simulink model "bms_final_sims_06"  (R2017b)
settings: Solver=VariableStepAuto  StartTime=0.0  StopTime=600  MaxStep=1e-4  RelTol=1e-3
undefined symbols (not defined in the file): DiscIntNeverNeededParam, Ion, Lithium, Ts_Control
libraries: powerlib x61, simulink x20, powerlib_meascontrol x3, simulink_extras x1, electricdrivelib x1
(part 1 of 2)
settings Model: SimulationMode=accelerator  Creator=Saagar  LastModifiedBy=student
settings OptimizationCC: EfficientMapNaN2IntZero=off
settings HardwareCC: TargetBitPerPointer=64  TargetBitPerSizeT=64  TargetBitPerPtrDiffT=64  TargetLongLongMode=on  TargetIntDivRoundTo=Zero  TargetEndianess=LittleEndian  TargetWordSize=64  TargetHWDeviceType=MATLAB Host  ProdEqTarget=off
settings CodeAppCC: MaxIdLength=128
settings GRTTargetCC: TargetLangStandard=C89/C90 (ANSI)  CombineOutputUpdateFcns=off  GRTInterface=on

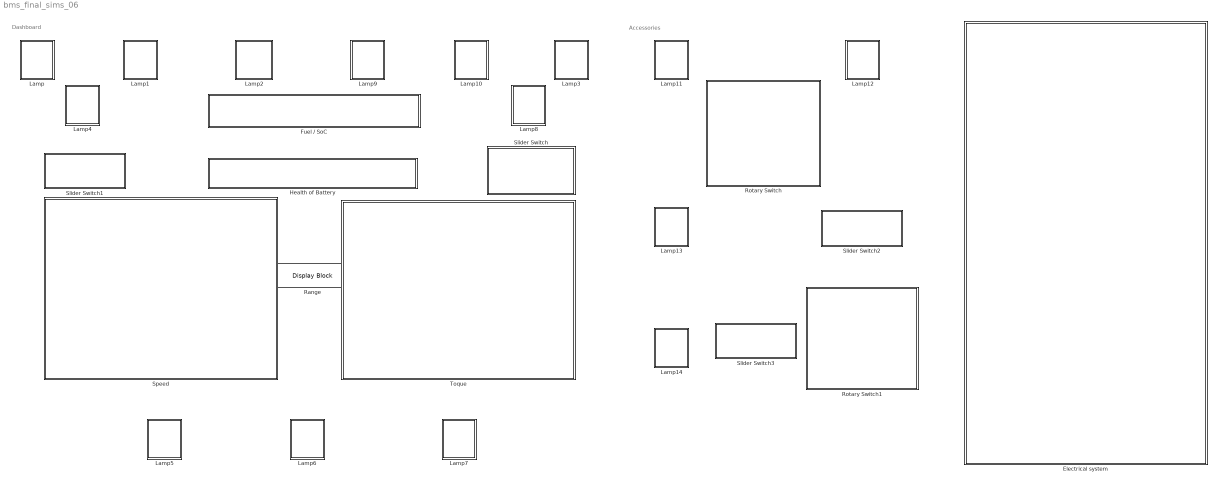
== system bms_final_sims_06 ==
  note: Accessories
  note: Dashboard
  Electrical system : Subsystem
  Fuel / SoC : Subsystem  DialogController=hmiCreateDDGDialog  IsWebBlock=on  mask(MWDashboardBlock){webBlockId=33162039-c99d-4f1a-a565-4d682c8cdccd, webBlockType=lineargauge, ShowInLibBrowser=on, ShowInitialText=on, HMISrcModelName=bms_final_sims_06}
      mask prompts: webBlockId "WebBlock Id"; webBlockType "WebBlock Type"; HMISrcModelName "Source Model"
      mask help: SimulinkHMI:dialogs:LinearGaugeDialogDesc
      mask Help: helpview([docroot '/mapfiles/simulink.map'], 'hmi_linear_gauge')
      mask Display:
      | if strcmp(get_param(bdroot(gcb),'BlockDiagramType'), 'library')
      |     image([(matlabroot) '/toolbox/simulink/hmi/icons/LinearGauge.png']);
      | end
  Health of Battery : Subsystem  DialogController=hmiCreateDDGDialog  IsWebBlock=on  mask(MWDashboardBlock){webBlockId=8809f0b6-5e37-4dfb-af47-87218bc99b36, webBlockType=lineargauge, ShowInLibBrowser=on, ShowInitialText=on, HMISrcModelName=bms_final_sims_06}
      mask prompts: webBlockId "WebBlock Id"; webBlockType "WebBlock Type"; HMISrcModelName "Source Model"
      mask help: SimulinkHMI:dialogs:LinearGaugeDialogDesc
      mask Help: helpview([docroot '/mapfiles/simulink.map'], 'hmi_linear_gauge')
      mask Display:
      | if strcmp(get_param(bdroot(gcb),'BlockDiagramType'), 'library')
      |     image([(matlabroot) '/toolbox/simulink/hmi/icons/LinearGauge.png']);
      | end
  Lamp : Subsystem  DialogController=hmiCreateDDGDialog  IsWebBlock=on  mask(MWDashboardBlock){webBlockId=60202423-3a17-48a5-95f7-77e0dff5e21e, webBlockType=lamp, ShowInLibBrowser=on, ShowInitialText=on, HMISrcModelName=bms_final_sims_06}
      mask prompts: webBlockType "WebBlock Type"; HMISrcModelName "Source Model"
      mask help: SimulinkHMI:dialogs:LampDialogDesc
      mask Help: helpview([docroot '/mapfiles/simulink.map'], 'hmi_lamp')
      mask Display:
      | if strcmp(get_param(bdroot(gcb),'BlockDiagramType'), 'library')
      |     image([(matlabroot) '/toolbox/simulink/hmi/icons/Lamp.png']);
      | end
  Lamp1 : Subsystem  DialogController=hmiCreateDDGDialog  IsWebBlock=on  mask(MWDashboardBlock){webBlockId=b772b617-bcd0-40f5-b9ce-808a282dbb2f, webBlockType=lamp, ShowInLibBrowser=on, ShowInitialText=on, HMISrcModelName=bms_final_sims_06}
      mask prompts: webBlockType "WebBlock Type"; HMISrcModelName "Source Model"
      mask help: SimulinkHMI:dialogs:LampDialogDesc
      mask Help: helpview([docroot '/mapfiles/simulink.map'], 'hmi_lamp')
      mask Display:
      | if strcmp(get_param(bdroot(gcb),'BlockDiagramType'), 'library')
      |     image([(matlabroot) '/toolbox/simulink/hmi/icons/Lamp.png']);
      | end
  Lamp10 : Subsystem  DialogController=hmiCreateDDGDialog  IsWebBlock=on  mask(MWDashboardBlock){webBlockId=5d6d0afe-77fe-451f-a78c-39b64214a0af, webBlockType=lamp, ShowInLibBrowser=on, ShowInitialText=on, HMISrcModelName=bms_final_sims_06}
      mask prompts: webBlockType "WebBlock Type"; HMISrcModelName "Source Model"
      mask help: SimulinkHMI:dialogs:LampDialogDesc
      mask Help: helpview([docroot '/mapfiles/simulink.map'], 'hmi_lamp')
      mask Display:
      | if strcmp(get_param(bdroot(gcb),'BlockDiagramType'), 'library')
      |     image([(matlabroot) '/toolbox/simulink/hmi/icons/Lamp.png']);
      | end
  Lamp11 : Subsystem  DialogController=hmiCreateDDGDialog  IsWebBlock=on  mask(MWDashboardBlock){webBlockId=0a72568f-0374-4cc2-9275-07ca00544e0d, webBlockType=lamp, ShowInLibBrowser=on, ShowInitialText=on, HMISrcModelName=bms_final_sims_06}
      mask prompts: webBlockType "WebBlock Type"; HMISrcModelName "Source Model"
      mask help: SimulinkHMI:dialogs:LampDialogDesc
      mask Help: helpview([docroot '/mapfiles/simulink.map'], 'hmi_lamp')
      mask Display:
      | if strcmp(get_param(bdroot(gcb),'BlockDiagramType'), 'library')
      |     image([(matlabroot) '/toolbox/simulink/hmi/icons/Lamp.png']);
      | end
  Lamp12 : Subsystem  DialogController=hmiCreateDDGDialog  IsWebBlock=on  mask(MWDashboardBlock){webBlockId=2b401852-71ce-442e-bb5f-6677ad9785ef, webBlockType=lamp, ShowInLibBrowser=on, ShowInitialText=on, HMISrcModelName=bms_final_sims_06}
      mask prompts: webBlockType "WebBlock Type"; HMISrcModelName "Source Model"
      mask help: SimulinkHMI:dialogs:LampDialogDesc
      mask Help: helpview([docroot '/mapfiles/simulink.map'], 'hmi_lamp')
      mask Display:
      | if strcmp(get_param(bdroot(gcb),'BlockDiagramType'), 'library')
      |     image([(matlabroot) '/toolbox/simulink/hmi/icons/Lamp.png']);
      | end
  Lamp13 : Subsystem  DialogController=hmiCreateDDGDialog  IsWebBlock=on  mask(MWDashboardBlock){webBlockId=2034ec30-c03c-420e-941b-856e970aeaa5, webBlockType=lamp, ShowInLibBrowser=on, ShowInitialText=on, HMISrcModelName=bms_final_sims_06}
      mask prompts: webBlockType "WebBlock Type"; HMISrcModelName "Source Model"
      mask help: SimulinkHMI:dialogs:LampDialogDesc
      mask Help: helpview([docroot '/mapfiles/simulink.map'], 'hmi_lamp')
      mask Display:
      | if strcmp(get_param(bdroot(gcb),'BlockDiagramType'), 'library')
      |     image([(matlabroot) '/toolbox/simulink/hmi/icons/Lamp.png']);
      | end
  Lamp14 : Subsystem  DialogController=hmiCreateDDGDialog  IsWebBlock=on  mask(MWDashboardBlock){webBlockId=15dee9ac-5ef9-4076-8e5a-31df19d47b6f, webBlockType=lamp, ShowInLibBrowser=on, ShowInitialText=on, HMISrcModelName=bms_final_sims_06}
      mask prompts: webBlockType "WebBlock Type"; HMISrcModelName "Source Model"
      mask help: SimulinkHMI:dialogs:LampDialogDesc
      mask Help: helpview([docroot '/mapfiles/simulink.map'], 'hmi_lamp')
      mask Display:
      | if strcmp(get_param(bdroot(gcb),'BlockDiagramType'), 'library')
      |     image([(matlabroot) '/toolbox/simulink/hmi/icons/Lamp.png']);
      | end
  Lamp2 : Subsystem  DialogController=hmiCreateDDGDialog  IsWebBlock=on  mask(MWDashboardBlock){webBlockId=89320668-7577-4891-bf3f-566db56929e4, webBlockType=lamp, ShowInLibBrowser=on, ShowInitialText=on, HMISrcModelName=bms_final_sims_06}
      mask prompts: webBlockType "WebBlock Type"; HMISrcModelName "Source Model"
      mask help: SimulinkHMI:dialogs:LampDialogDesc
      mask Help: helpview([docroot '/mapfiles/simulink.map'], 'hmi_lamp')
      mask Display:
      | if strcmp(get_param(bdroot(gcb),'BlockDiagramType'), 'library')
      |     image([(matlabroot) '/toolbox/simulink/hmi/icons/Lamp.png']);
      | end
  Lamp3 : Subsystem  DialogController=hmiCreateDDGDialog  IsWebBlock=on  mask(MWDashboardBlock){webBlockId=b6a86ebd-c106-4c49-970d-cc15b3a46232, webBlockType=lamp, ShowInLibBrowser=on, ShowInitialText=on, HMISrcModelName=bms_final_sims_06}
      mask prompts: webBlockType "WebBlock Type"; HMISrcModelName "Source Model"
      mask help: SimulinkHMI:dialogs:LampDialogDesc
      mask Help: helpview([docroot '/mapfiles/simulink.map'], 'hmi_lamp')
      mask Display:
      | if strcmp(get_param(bdroot(gcb),'BlockDiagramType'), 'library')
      |     image([(matlabroot) '/toolbox/simulink/hmi/icons/Lamp.png']);
      | end
  Lamp4 : Subsystem  DialogController=hmiCreateDDGDialog  IsWebBlock=on  mask(MWDashboardBlock){webBlockId=844a4c6a-a02b-48df-b256-6a68b1dbece4, webBlockType=lamp, ShowInLibBrowser=on, ShowInitialText=on, HMISrcModelName=bms_final_sims_06}
      mask prompts: webBlockType "WebBlock Type"; HMISrcModelName "Source Model"
      mask help: SimulinkHMI:dialogs:LampDialogDesc
      mask Help: helpview([docroot '/mapfiles/simulink.map'], 'hmi_lamp')
      mask Display:
      | if strcmp(get_param(bdroot(gcb),'BlockDiagramType'), 'library')
      |     image([(matlabroot) '/toolbox/simulink/hmi/icons/Lamp.png']);
      | end
  Lamp5 : Subsystem  DialogController=hmiCreateDDGDialog  IsWebBlock=on  mask(MWDashboardBlock){webBlockId=11f2fa90-eb2a-4fe6-8dd8-94244659f303, webBlockType=lamp, ShowInLibBrowser=on, ShowInitialText=on, HMISrcModelName=bms_final_sims_06}
      mask prompts: webBlockType "WebBlock Type"; HMISrcModelName "Source Model"
      mask help: SimulinkHMI:dialogs:LampDialogDesc
      mask Help: helpview([docroot '/mapfiles/simulink.map'], 'hmi_lamp')
      mask Display:
      | if strcmp(get_param(bdroot(gcb),'BlockDiagramType'), 'library')
      |     image([(matlabroot) '/toolbox/simulink/hmi/icons/Lamp.png']);
      | end
  Lamp6 : Subsystem  DialogController=hmiCreateDDGDialog  IsWebBlock=on  mask(MWDashboardBlock){webBlockId=ab68f173-faf5-42a8-b25f-7a197262fa87, webBlockType=lamp, ShowInLibBrowser=on, ShowInitialText=on, HMISrcModelName=bms_final_sims_06}
      mask prompts: webBlockType "WebBlock Type"; HMISrcModelName "Source Model"
      mask help: SimulinkHMI:dialogs:LampDialogDesc
      mask Help: helpview([docroot '/mapfiles/simulink.map'], 'hmi_lamp')
      mask Display:
      | if strcmp(get_param(bdroot(gcb),'BlockDiagramType'), 'library')
      |     image([(matlabroot) '/toolbox/simulink/hmi/icons/Lamp.png']);
      | end
  Lamp7 : Subsystem  DialogController=hmiCreateDDGDialog  IsWebBlock=on  mask(MWDashboardBlock){webBlockId=81e08fe1-4f2d-481f-ba0b-4bb12e2dc645, webBlockType=lamp, ShowInLibBrowser=on, ShowInitialText=on, HMISrcModelName=bms_final_sims_06}
      mask prompts: webBlockType "WebBlock Type"; HMISrcModelName "Source Model"
      mask help: SimulinkHMI:dialogs:LampDialogDesc
      mask Help: helpview([docroot '/mapfiles/simulink.map'], 'hmi_lamp')
      mask Display:
      | if strcmp(get_param(bdroot(gcb),'BlockDiagramType'), 'library')
      |     image([(matlabroot) '/toolbox/simulink/hmi/icons/Lamp.png']);
      | end
  Lamp8 : Subsystem  DialogController=hmiCreateDDGDialog  IsWebBlock=on  mask(MWDashboardBlock){webBlockId=6ab1c72b-15eb-4bf1-ab8d-4a746cbd358c, webBlockType=lamp, ShowInLibBrowser=on, ShowInitialText=on, HMISrcModelName=bms_final_sims_06}
      mask prompts: webBlockType "WebBlock Type"; HMISrcModelName "Source Model"
      mask help: SimulinkHMI:dialogs:LampDialogDesc
      mask Help: helpview([docroot '/mapfiles/simulink.map'], 'hmi_lamp')
      mask Display:
      | if strcmp(get_param(bdroot(gcb),'BlockDiagramType'), 'library')
      |     image([(matlabroot) '/toolbox/simulink/hmi/icons/Lamp.png']);
      | end
  Lamp9 : Subsystem  DialogController=hmiCreateDDGDialog  IsWebBlock=on  mask(MWDashboardBlock){webBlockId=3f2b2ded-00af-4410-9f91-19541f575b1a, webBlockType=lamp, ShowInLibBrowser=on, ShowInitialText=on, HMISrcModelName=bms_final_sims_06}
      mask prompts: webBlockType "WebBlock Type"; HMISrcModelName "Source Model"
      mask help: SimulinkHMI:dialogs:LampDialogDesc
      mask Help: helpview([docroot '/mapfiles/simulink.map'], 'hmi_lamp')
      mask Display:
      | if strcmp(get_param(bdroot(gcb),'BlockDiagramType'), 'library')
      |     image([(matlabroot) '/toolbox/simulink/hmi/icons/Lamp.png']);
      | end
  Range : DisplayBlock  WebBlockId=824  ModelName=bms_final_sims_06  LabelPosition=Hide  ShowInitialText=on  ShowFormattedStrings=off  Format=long  Alignment=Center
  Rotary Switch : Subsystem  DialogController=hmiCreateDDGDialog  IsWebBlock=on  mask(MWDashboardBlock){webBlockId=4826fd6e-fb06-4944-a463-9540ffd16b42, webBlockType=discreteknob, ShowInLibBrowser=on, ShowInitialText=on, HMISrcModelName=bms_final_sims_06}
      mask prompts: webBlockId "WebBlock Id"; webBlockType "WebBlock Type"; HMISrcModelName "Source Model"
      mask help: SimulinkHMI:dialogs:DiscreteKnobDialogDesc
      mask Help: helpview([docroot '/mapfiles/simulink.map'], 'hmi_rotary_switch')
      mask Display:
      | model = bdroot(gcb);
      | if strcmp(get_param(model,'BlockDiagramType'), 'library')
      |     image([(matlabroot) '/toolbox/simulink/hmi/icons/DiscreteKnob.png']);
      | end
  Rotary Switch1 : Subsystem  DialogController=hmiCreateDDGDialog  IsWebBlock=on  mask(MWDashboardBlock){webBlockId=004f83a7-65e5-41a6-9793-17691810caf2, webBlockType=discreteknob, ShowInLibBrowser=on, ShowInitialText=on, HMISrcModelName=bms_final_sims_06}
      mask prompts: webBlockId "WebBlock Id"; webBlockType "WebBlock Type"; HMISrcModelName "Source Model"
      mask help: SimulinkHMI:dialogs:DiscreteKnobDialogDesc
      mask Help: helpview([docroot '/mapfiles/simulink.map'], 'hmi_rotary_switch')
      mask Display:
      | model = bdroot(gcb);
      | if strcmp(get_param(model,'BlockDiagramType'), 'library')
      |     image([(matlabroot) '/toolbox/simulink/hmi/icons/DiscreteKnob.png']);
      | end
  Slider Switch : Subsystem  DialogController=hmiCreateDDGDialog  IsWebBlock=on  mask(MWDashboardBlock){webBlockId=b33d24b0-9713-4f3a-b907-0250ae95ad7b, webBlockType=sliderswitch, ShowInLibBrowser=on, ShowInitialText=on, HMISrcModelName=bms_final_sims_06}
      mask prompts: webBlockId "WebBlock Id"; webBlockType "WebBlock Type"; HMISrcModelName "Source Model"
      mask help: SimulinkHMI:dialogs:SwitchDialogDesc
      mask Help: helpview([docroot '/mapfiles/simulink.map'], 'hmi_slider_switch')
      mask Display:
      | if strcmp(get_param(bdroot(gcb),'BlockDiagramType'), 'library')
      |     image([(matlabroot) '/toolbox/simulink/hmi/icons/SliderSwitch.png']);
      | end
  Slider Switch1 : Subsystem  DialogController=hmiCreateDDGDialog  IsWebBlock=on  mask(MWDashboardBlock){webBlockId=e75f6dc5-ab5c-4d7d-beb3-4e0f2ef2dcf0, webBlockType=sliderswitch, ShowInLibBrowser=on, ShowInitialText=on, HMISrcModelName=bms_final_sims_06}
      mask prompts: webBlockId "WebBlock Id"; webBlockType "WebBlock Type"; HMISrcModelName "Source Model"
      mask help: SimulinkHMI:dialogs:SwitchDialogDesc
      mask Help: helpview([docroot '/mapfiles/simulink.map'], 'hmi_slider_switch')
      mask Display:
      | if strcmp(get_param(bdroot(gcb),'BlockDiagramType'), 'library')
      |     image([(matlabroot) '/toolbox/simulink/hmi/icons/SliderSwitch.png']);
      | end
  Slider Switch2 : Subsystem  DialogController=hmiCreateDDGDialog  IsWebBlock=on  mask(MWDashboardBlock){webBlockId=6e0caa40-7a6a-4072-b1f3-4d53d29c6100, webBlockType=sliderswitch, ShowInLibBrowser=on, ShowInitialText=on, HMISrcModelName=bms_final_sims_06}
      mask prompts: webBlockId "WebBlock Id"; webBlockType "WebBlock Type"; HMISrcModelName "Source Model"
      mask help: SimulinkHMI:dialogs:SwitchDialogDesc
      mask Help: helpview([docroot '/mapfiles/simulink.map'], 'hmi_slider_switch')
      mask Display:
      | if strcmp(get_param(bdroot(gcb),'BlockDiagramType'), 'library')
      |     image([(matlabroot) '/toolbox/simulink/hmi/icons/SliderSwitch.png']);
      | end
  Slider Switch3 : Subsystem  DialogController=hmiCreateDDGDialog  IsWebBlock=on  mask(MWDashboardBlock){webBlockId=17662730-6830-47a9-b1c0-e2f214473cb4, webBlockType=sliderswitch, ShowInLibBrowser=on, ShowInitialText=on, HMISrcModelName=bms_final_sims_06}
      mask prompts: webBlockId "WebBlock Id"; webBlockType "WebBlock Type"; HMISrcModelName "Source Model"
      mask help: SimulinkHMI:dialogs:SwitchDialogDesc
      mask Help: helpview([docroot '/mapfiles/simulink.map'], 'hmi_slider_switch')
      mask Display:
      | if strcmp(get_param(bdroot(gcb),'BlockDiagramType'), 'library')
      |     image([(matlabroot) '/toolbox/simulink/hmi/icons/SliderSwitch.png']);
      | end
  Speed : Subsystem  DialogController=hmiCreateDDGDialog  IsWebBlock=on  mask(MWDashboardBlock){webBlockId=f8eab75d-284a-4f52-aea2-2470c4576d66, webBlockType=circulargauge, ShowInLibBrowser=on, ShowInitialText=on, HMISrcModelName=bms_final_sims_06}
      mask prompts: webBlockId "WebBlock Id"; webBlockType "WebBlock Type"; HMISrcModelName "Source Model"
      mask help: SimulinkHMI:dialogs:CircularGaugeDialogDesc
      mask Help: helpview([docroot '/mapfiles/simulink.map'], 'hmi_gauge')
      mask Display:
      | if strcmp(get_param(bdroot(gcb),'BlockDiagramType'), 'library')
      |     image([(matlabroot) '/toolbox/simulink/hmi/icons/CircularGauge.png']);
      | end
  Toque : Subsystem  DialogController=hmiCreateDDGDialog  IsWebBlock=on  mask(MWDashboardBlock){webBlockId=3de0aea9-e842-4bc1-a604-82e06c8cc4e5, webBlockType=circulargauge, ShowInLibBrowser=on, ShowInitialText=on, HMISrcModelName=bms_final_sims_06}
      mask prompts: webBlockId "WebBlock Id"; webBlockType "WebBlock Type"; HMISrcModelName "Source Model"
      mask help: SimulinkHMI:dialogs:CircularGaugeDialogDesc
      mask Help: helpview([docroot '/mapfiles/simulink.map'], 'hmi_gauge')
      mask Display:
      | if strcmp(get_param(bdroot(gcb),'BlockDiagramType'), 'library')
      |     image([(matlabroot) '/toolbox/simulink/hmi/icons/CircularGauge.png']);
      | end

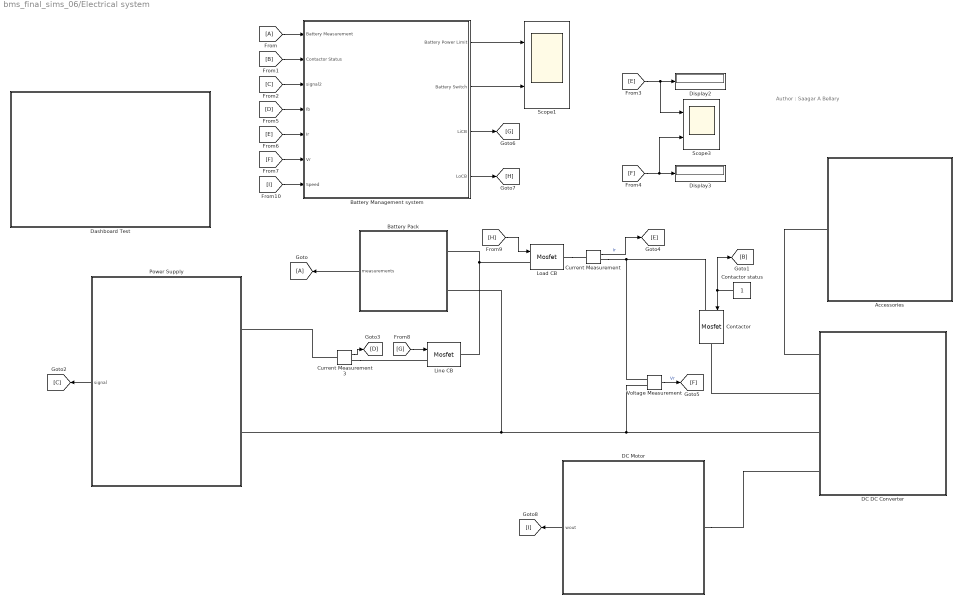
== system bms_final_sims_06/Electrical system ==
  note: Author : Saagar A Bellary
  Accessories : Subsystem
      mask Display: image('accessories.jpg')
  Battery Management system : Subsystem
      mask Display: image('BMS.jpg')
  Battery Pack : Subsystem  mask{NomV=48, NomQ=100, SOC=62.32, t=[0, 500, 1000 1500  2000 2500], e=[27, 32, 27  20  10 0], RisingSlewLimit=0.5, FallingSlewLimit=-0.5}
      mask prompts: NomV "Nominal voltage (V)"; NomQ "Rated capacity (Ah)"; SOC "Initial state-of-charge (%)"; t "Time (s):"; e "Ambient Temparature"; RisingSlewLimit "Simulink:blkprm_prompts:RateLimRisingSlewRate"; FallingSlewLimit "Simulink:blkprm_prompts:RateLimFallingSlewRate"
      mask TypeOptions NomV: Battery Pack/NomV
      mask TypeOptions NomQ: Battery Pack/NomQ
      mask TypeOptions SOC: Battery Pack/SOC
      mask TypeOptions t: Ambient Temperature/t
      mask TypeOptions e: Ambient Temperature/e
      mask TypeOptions RisingSlewLimit: 6 oC//min/RisingSlewLimit
      mask TypeOptions FallingSlewLimit: 6 oC//min/FallingSlewLimit
      mask DialogControl RisingSlewLimit Prompt: Rising slew rate:
      mask DialogControl FallingSlewLimit Prompt: Falling slew rate:
      mask Display: image('Battery.jpg')
  Contactor : powerlib/Power Electronics/Mosfet  Ron=0.01  Lon=0  Rd=0.01  Vfd=0  IC=0  Rs=1e9  Cs=inf  Measurements=off
  Contactor status : Constant
  Current Measurement : powerlib/Measurements/Current Measurement  PhasorSimulation=off  OutputType=Complex  PSBequivalent=0
  Current Measurement3 : powerlib/Measurements/Current Measurement  PhasorSimulation=off  OutputType=Complex  PSBequivalent=0
  DC DC Converter : Subsystem  mask{Value=0.75, Fsw=20e3, Ts=0, Inductance=0.152e-03, Capacitance=4700e-06}
      mask prompts: Value "Duty Ratio"; Fsw "Switching frequency (Hz):"; Ts "Sample time:"; Inductance "Inductance (H):"; Capacitance "Capacitance (F):"
      mask TypeOptions Value: D/Value
      mask TypeOptions Fsw:
      | PWM Generator
      | (DC-DC)/Fsw
      mask TypeOptions Ts:
      | PWM Generator
      | (DC-DC)/Ts
      mask TypeOptions Inductance: LB1/Inductance
      mask TypeOptions Capacitance: CB1/Capacitance
      mask Display: image('DCDC.jpg')
  DC Motor : Subsystem  mask{Amplitude=110}
      mask prompts: Amplitude "Field Voltage (V):"
      mask TypeOptions Amplitude: Ef/Amplitude
      mask Display: image('Motor.jpg')
  Dashboard Test : Subsystem
      mask Display: image('dashboard.jpg')
  Display2 : Display
  Display3 : Display
  Line CB : powerlib/Power Electronics/Mosfet  Ron=0.01  Lon=0  Rd=0.01  Vfd=0  IC=0  Rs=1e9  Cs=inf  Measurements=off
  Load CB : powerlib/Power Electronics/Mosfet  Ron=0.01  Lon=0  Rd=0.01  Vfd=0  IC=0  Rs=1e9  Cs=inf  Measurements=off
  Power Supply : Subsystem  mask{Value=54, Capacitance=4700e-6, Inductance=100e-6, Inductance1=10e-6}
      mask prompts: Value "Battery Voltage Max(V)"; Capacitance "Output Capacitance (F):"; Inductance "Primary Inductance (H):"; Inductance1 "Secondary Inductance (H):"
      mask TypeOptions Value: Vref/Value
      mask TypeOptions Capacitance: Co/Capacitance
      mask TypeOptions Inductance: Lo1/Inductance
      mask TypeOptions Inductance1: Lo2/Inductance
      mask Display: image('supply.jpg')
  Scope1 : Scope  NumInputPorts=2
  Scope3 : Scope  NumInputPorts=2
  Voltage Measurement : powerlib/Measurements/Voltage Measurement  PhasorSimulation=off  OutputType=Complex  PSBequivalent=0
  wires:
  Contactor status/1 -> [B], Contactor/1
  Battery Management system/2(Battery Switch) -> Scope1/2
  Battery Management system/1("Battery Power Limit ") -> Scope1/1
  [E] -> Scope3/1, Display2/1
  [F] -> Display3/1, Scope3/2
  [B] -> Battery Management system/2(Contactor Status)
  [A] -> Battery Management system/1(Battery Measurement)
  [C] -> Battery Management system/3(signal2)
  [D] -> Battery Management system/4(Ib)
  [E] -> Battery Management system/5(Ir)
  [F] -> Battery Management system/6("Vr ")
  Battery Management system/3(LiCB) -> [G]
  Battery Management system/4(LoCB) -> [H]
  Battery Pack/1("measurements ") -> [A]
  Power Supply/1(signal) -> [C]
  Current Measurement3/1 -> [D]
  Voltage Measurement/1 -> [F]  "Vr"
  Current Measurement/1 -> [E]  "Ir"
  [G] -> Line CB/1
  [H] -> Load CB/1
  DC Motor/1(wout) -> [I]
  [I] -> Battery Management system/7(Speed)
  connections:
  Load CB/RConn1 -- Current Measurement/LConn1
  Current Measurement/RConn1 -- Voltage Measurement/LConn1 -- Contactor/LConn1
  Load CB/LConn1 -- Line CB/RConn1 -- Battery Pack/LConn1
  DC DC Converter/LConn3 -- Battery Pack/LConn2 -- Power Supply/LConn2 -- Voltage Measurement/LConn2
  DC Motor/LConn1 -- DC DC Converter/LConn4
  DC DC Converter/LConn2 -- Contactor/RConn1
  DC DC Converter/LConn1 -- Accessories/LConn1
  Current Measurement3/LConn1 -- Power Supply/LConn1
  Current Measurement3/RConn1 -- Line CB/LConn1

== system bms_final_sims_06/Fuel // SoC ==

== system bms_final_sims_06/Health of Battery ==

== system bms_final_sims_06/Lamp ==

== system bms_final_sims_06/Lamp1 ==

== system bms_final_sims_06/Lamp10 ==

== system bms_final_sims_06/Lamp11 ==

== system bms_final_sims_06/Lamp12 ==

== system bms_final_sims_06/Lamp13 ==

== system bms_final_sims_06/Lamp14 ==

== system bms_final_sims_06/Lamp2 ==

== system bms_final_sims_06/Lamp3 ==

== system bms_final_sims_06/Lamp4 ==

== system bms_final_sims_06/Lamp5 ==

== system bms_final_sims_06/Lamp6 ==

== system bms_final_sims_06/Lamp7 ==

== system bms_final_sims_06/Lamp8 ==

== system bms_final_sims_06/Lamp9 ==

== system bms_final_sims_06/Rotary Switch ==

== system bms_final_sims_06/Rotary Switch1 ==

== system bms_final_sims_06/Slider Switch ==

== system bms_final_sims_06/Slider Switch1 ==

== system bms_final_sims_06/Slider Switch2 ==

== system bms_final_sims_06/Slider Switch3 ==

== system bms_final_sims_06/Speed ==

== system bms_final_sims_06/Toque ==

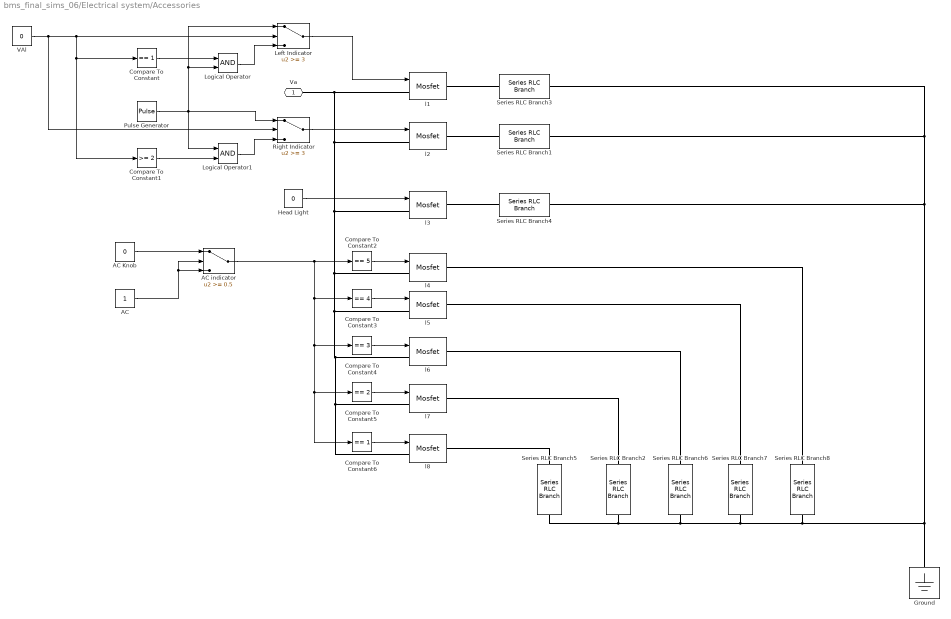
== system bms_final_sims_06/Electrical system/Accessories ==
  AC : Constant
  AC Knob : Constant  Value=0
  AC indicator : Switch  Threshold=0.5
  Compare To Constant : simulink/Logic and Bit Operations/Compare To Constant  relop===  const=1  OutDataTypeStr=boolean
  Compare To Constant1 : simulink/Logic and Bit Operations/Compare To Constant  relop=>=  const=2  OutDataTypeStr=boolean
  Compare To Constant2 : simulink/Logic and Bit Operations/Compare To Constant  relop===  const=5  OutDataTypeStr=boolean
  Compare To Constant3 : simulink/Logic and Bit Operations/Compare To Constant  relop===  const=4  OutDataTypeStr=boolean
  Compare To Constant4 : simulink/Logic and Bit Operations/Compare To Constant  relop===  const=3  OutDataTypeStr=boolean
  Compare To Constant5 : simulink/Logic and Bit Operations/Compare To Constant  relop===  const=2  OutDataTypeStr=boolean
  Compare To Constant6 : simulink/Logic and Bit Operations/Compare To Constant  relop===  const=1  OutDataTypeStr=boolean
  Ground : powerlib/Elements/Ground  LConnTagsString=a
  Head Light : Constant  Value=0
  Left Indicator : Switch  Threshold=3
  Logical Operator : Logic  AllPortsSameDT=off  OutDataTypeStr=boolean
  Logical Operator1 : Logic  AllPortsSameDT=off  OutDataTypeStr=boolean
  Pulse Generator : DiscretePulseGenerator  PulseType=Time based  Period=0.5  PulseWidth=50
  Right Indicator : Switch  Threshold=3
  Series RLC Branch1 : powerlib/Elements/Series RLC Branch  LConnTagsString=__new0  RConnTagsString=__new0  BranchType=R  Resistance=20  Inductance=0.152e-03  SetiL0=off  InitialCurrent=0  Capacitance=0  Setx0=off  InitialVoltage=0  Measurements=None
  Series RLC Branch2 : powerlib/Elements/Series RLC Branch  LConnTagsString=__new0  RConnTagsString=__new0  BranchType=R  Resistance=9  Inductance=0.152e-03  SetiL0=off  InitialCurrent=0  Capacitance=0  Setx0=off  InitialVoltage=0  Measurements=None
  Series RLC Branch3 : powerlib/Elements/Series RLC Branch  LConnTagsString=__new0  RConnTagsString=__new0  BranchType=R  Resistance=20  Inductance=0.152e-03  SetiL0=off  InitialCurrent=0  Capacitance=0  Setx0=off  InitialVoltage=0  Measurements=None
  Series RLC Branch4 : powerlib/Elements/Series RLC Branch  LConnTagsString=__new0  RConnTagsString=__new0  BranchType=R  Resistance=12.5  Inductance=0.152e-03  SetiL0=off  InitialCurrent=0  Capacitance=0  Setx0=off  InitialVoltage=0  Measurements=None
  Series RLC Branch5 : powerlib/Elements/Series RLC Branch  LConnTagsString=__new0  RConnTagsString=__new0  BranchType=R  Resistance=12  Inductance=0.152e-03  SetiL0=off  InitialCurrent=0  Capacitance=0  Setx0=off  InitialVoltage=0  Measurements=None
  Series RLC Branch6 : powerlib/Elements/Series RLC Branch  LConnTagsString=__new0  RConnTagsString=__new0  BranchType=R  Resistance=7.5  Inductance=0.152e-03  SetiL0=off  InitialCurrent=0  Capacitance=0  Setx0=off  InitialVoltage=0  Measurements=None
  Series RLC Branch7 : powerlib/Elements/Series RLC Branch  LConnTagsString=__new0  RConnTagsString=__new0  BranchType=R  Resistance=6  Inductance=0.152e-03  SetiL0=off  InitialCurrent=0  Capacitance=0  Setx0=off  InitialVoltage=0  Measurements=None
  Series RLC Branch8 : powerlib/Elements/Series RLC Branch  LConnTagsString=__new0  RConnTagsString=__new0  BranchType=R  Resistance=4.5  Inductance=0.152e-03  SetiL0=off  InitialCurrent=0  Capacitance=0  Setx0=off  InitialVoltage=0  Measurements=None
  "VAl " : Constant  Value=0
  l1 : powerlib/Power Electronics/Mosfet  Ron=0.01  Lon=0  Rd=0.01  Vfd=0  IC=0  Rs=1e9  Cs=inf  Measurements=off
  l2 : powerlib/Power Electronics/Mosfet  Ron=0.01  Lon=0  Rd=0.01  Vfd=0  IC=0  Rs=1e9  Cs=inf  Measurements=off
  l3 : powerlib/Power Electronics/Mosfet  Ron=0.01  Lon=0  Rd=0.01  Vfd=0  IC=0  Rs=1e9  Cs=inf  Measurements=off
  l{4..8} (5 alike) : powerlib/Power Electronics/Mosfet  Ron=0.01  Lon=0  Rd=0.01  Vfd=1  IC=0  Rs=1e9  Cs=inf  Measurements=off
  Va : PMIOPort  Port=1  Side=Left
  wires:
  Head Light/1 -> l3/1
  "VAl "/1 -> Right Indicator/2, Compare To Constant1/1, Compare To Constant/1, Left Indicator/2
  Pulse Generator/1 -> Right Indicator/1, Logical Operator/2, Left Indicator/1, Logical Operator1/1
  Right Indicator/1 -> l2/1
  Left Indicator/1 -> l1/1
  AC/1 -> AC indicator/2, AC indicator/3
  AC Knob/1 -> AC indicator/1
  Compare To Constant2/1 -> l4/1
  Compare To Constant3/1 -> l5/1
  Compare To Constant4/1 -> l6/1
  Compare To Constant5/1 -> l7/1
  Compare To Constant6/1 -> l8/1
  AC indicator/1 -> Compare To Constant3/1, Compare To Constant4/1, Compare To Constant5/1, Compare To Constant6/1, Compare To Constant2/1
  Logical Operator/1 -> Left Indicator/3
  Compare To Constant/1 -> Logical Operator/1
  Compare To Constant1/1 -> Logical Operator1/2
  Logical Operator1/1 -> Right Indicator/3
  connections:
  l2/RConn1 -- Series RLC Branch1/LConn1
  l3/RConn1 -- Series RLC Branch4/LConn1
  l1/LConn1 -- l7/LConn1 -- l8/LConn1 -- l6/LConn1 -- l5/LConn1 -- l4/LConn1 -- l3/LConn1 -- l2/LConn1 -- Va/RConn1
  l1/RConn1 -- Series RLC Branch3/LConn1
  Series RLC Branch4/RConn1 -- Series RLC Branch5/RConn1 -- Series RLC Branch2/RConn1 -- Series RLC Branch6/RConn1 -- Series RLC Branch7/RConn1 -- Series RLC Branch8/RConn1 -- Ground/LConn1 -- Series RLC Branch1/RConn1 -- Series RLC Branch3/RConn1
  Series RLC Branch5/LConn1 -- l8/RConn1
  Series RLC Branch2/LConn1 -- l7/RConn1
  Series RLC Branch6/LConn1 -- l6/RConn1
  Series RLC Branch7/LConn1 -- l5/RConn1
  Series RLC Branch8/LConn1 -- l4/RConn1

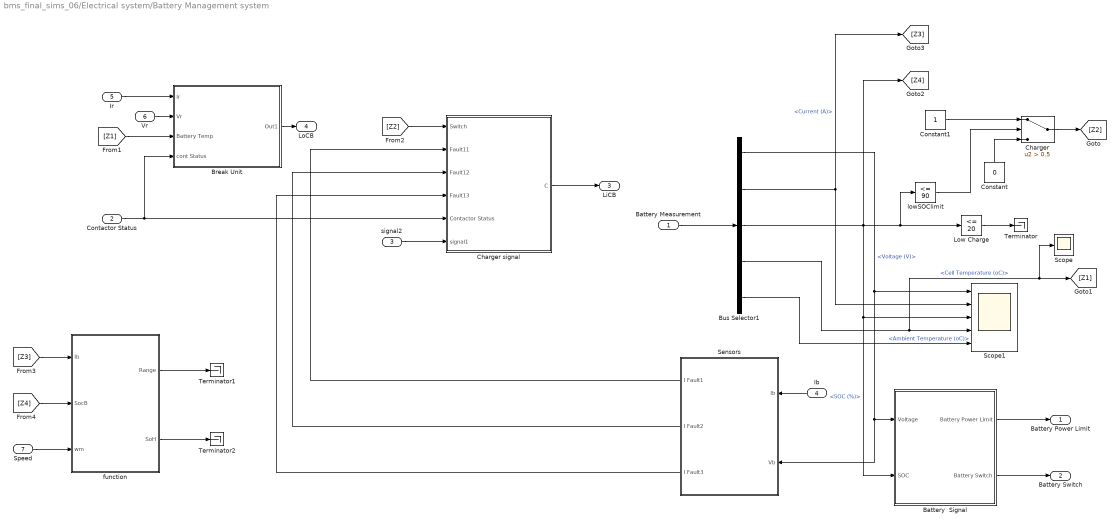
== system bms_final_sims_06/Electrical system/Battery Management system ==
  Battery Measurement : Inport
  Contactor Status : Inport  Port=2
  signal2 : Inport  Port=3
  Ib : Inport  Port=4
  Ir : Inport  Port=5
  "Vr " : Inport  Port=6
  Speed : Inport  Port=7
  " function" : Subsystem
  Battery  Signal : Subsystem
  Break Unit : Subsystem
  Bus Selector1 : BusSelector  OutputSignals=Voltage (V),Current (A),SOC (%),Cell Temperature (oC),Ambient Temperature (oC)
  Charger : Switch  Criteria=u2 > Threshold  Threshold=0.5
  Charger signal : Subsystem
  Constant : Constant  Value=0
  Constant1 : Constant
  Low Charge : simulink/Logic and Bit Operations/Compare To Constant  relop=<=  const=20  OutDataTypeStr=boolean
  Scope : Scope
  Scope1 : Scope  NumInputPorts=5
  Sensors : Subsystem
  Terminator : Terminator
  Terminator1 : Terminator
  Terminator2 : Terminator
  lowSOClimit : simulink/Logic and Bit Operations/Compare To Constant  relop=<=  const=90  OutDataTypeStr=boolean
  "Battery Power Limit " : Outport
  Battery Switch : Outport  Port=2
  LiCB : Outport  Port=3
  LoCB : Outport  Port=4
  wires:
  Battery  Signal/1("Battery Power Limit ") -> "Battery Power Limit "/1
  Battery  Signal/2(Battery Switch) -> Battery Switch/1
  Bus Selector1/2 -> [Z3], Scope1/2  "<Current (A)>"
  Battery Measurement/1 -> Bus Selector1/1
  lowSOClimit/1 -> Charger/2
  Constant/1 -> Charger/3
  Charger signal/1(C) -> LiCB/1
  Constant1/1 -> Charger/1
  Sensors/1(I Fault1) -> Charger signal/2(Fault11)
  Sensors/2(I Fault2) -> Charger signal/3(Fault12)
  Sensors/3(I Fault3) -> Charger signal/4(Fault13)
  Bus Selector1/4 -> [Z1], Scope/1, Scope1/4  "<Cell Temperature (oC)>"
  Bus Selector1/1 -> Battery  Signal/1(Voltage), Sensors/2(Vb), Scope1/1  "<Voltage (V)>"
  Bus Selector1/3 -> [Z4], Scope1/3, Battery  Signal/2(SOC), Low Charge/1, lowSOClimit/1  "<SOC (%)>"
  Bus Selector1/5 -> Scope1/5  "<Ambient Temperature (oC)>"
  Low Charge/1 -> Terminator/1
  Ib/1 -> Sensors/1(Ib)
  signal2/1 -> Charger signal/6(signal1)
  [Z1] -> Break Unit/3(Battery Temp)
  Contactor Status/1 -> Break Unit/4("cont Status "), Charger signal/5(Contactor Status)
  Break Unit/1(Out1) -> LoCB/1
  Ir/1 -> Break Unit/1(Ir)
  "Vr "/1 -> Break Unit/2(Vr)
  Charger/1 -> [Z2]
  [Z2] -> Charger signal/1(Switch)
  [Z3] -> " function"/1(Ib)
  [Z4] -> " function"/2(SocB)
  " function"/1(Range) -> Terminator1/1
  " function"/2(SoH) -> Terminator2/1
  Speed/1 -> " function"/3(wm)

== system bms_final_sims_06/Electrical system/Battery Pack ==
  6 oC/min : RateLimiter  RisingSlewLimit=RisingSlewLimit  FallingSlewLimit=FallingSlewLimit  SampleTimeMode=inherited
  Ambient Temperature : powerlib_meascontrol/Pulse & Signal Generators/Stair Generator  t=t  e=e  Ts=0
      settings: SourceProductName=Simscape Power Systems
  Battery Cell Equivalent : Subsystem
      mask Display: image('cell.jpg');
  +B : PMIOPort  Port=1  Side=Left
  -B : PMIOPort  Port=2  Side=Left
  "measurements " : Outport
  wires:
  Ambient Temperature/1 -> 6 oC/min/1
  6 oC/min/1 -> Battery Cell Equivalent/1(t)
  Battery Cell Equivalent/1(M) -> "measurements "/1
  connections:
  Battery Cell Equivalent/LConn1 -- +B/RConn1
  Battery Cell Equivalent/LConn2 -- -B/RConn1

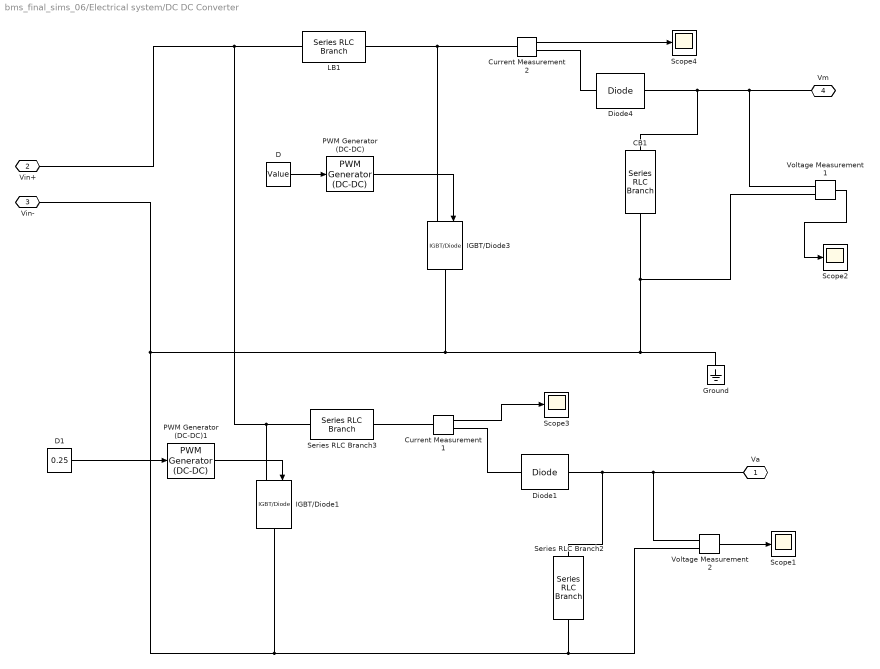
== system bms_final_sims_06/Electrical system/DC DC Converter ==
  CB1 : powerlib/Elements/Series RLC Branch  LConnTagsString=__new0  RConnTagsString=__new0  BranchType=C  Resistance=0  Inductance=0  SetiL0=off  InitialCurrent=0  Capacitance=Capacitance  Setx0=off  InitialVoltage=0  Measurements=None
  Current Measurement1 : powerlib/Measurements/Current Measurement  PhasorSimulation=off  OutputType=Complex  PSBequivalent=0
  Current Measurement2 : powerlib/Measurements/Current Measurement  PhasorSimulation=off  OutputType=Complex  PSBequivalent=0
  D : Constant  Value=Value
  D1 : Constant  Value=0.25
  Diode1 : powerlib/Power Electronics/Diode  Ron=0.001  Lon=0  Vf=0.8  IC=0  UseSnubber=off  Rs=500  Cs=250e-9  Measurements=off
  Diode4 : powerlib/Power Electronics/Diode  Ron=0.001  Lon=0  Vf=0.8  IC=0  UseSnubber=off  Rs=500  Cs=250e-9  Measurements=off
  Ground : powerlib/Elements/Ground  LConnTagsString=a
  IGBT/Diode1 : powerlib/Power Electronics/IGBT//Diode  Ron=1e-3  Rs=1e5  Cs=inf  Measurements=off
  IGBT/Diode3 : powerlib/Power Electronics/IGBT//Diode  Ron=1e-3  Rs=1e5  Cs=inf  Measurements=off
  LB1 : powerlib/Elements/Series RLC Branch  LConnTagsString=__new0  RConnTagsString=__new0  BranchType=L  Resistance=0  Inductance=Inductance  SetiL0=off  InitialCurrent=0  Capacitance=0  Setx0=off  InitialVoltage=0  Measurements=None
  PWM Generator (DC-DC) : powerlib_meascontrol/Pulse & Signal Generators/PWM Generator (DC-DC)  Fsw=Fsw  Ts=Ts
  PWM Generator (DC-DC)1 : powerlib_meascontrol/Pulse & Signal Generators/PWM Generator (DC-DC)  Fsw=20e3  Ts=0
  Scope{1..4} (4 alike) : Scope
  Series RLC Branch2 : powerlib/Elements/Series RLC Branch  LConnTagsString=__new0  RConnTagsString=__new0  BranchType=C  Resistance=0  Inductance=0  SetiL0=off  InitialCurrent=0  Capacitance=4700e-06  Setx0=off  InitialVoltage=0  Measurements=None
  Series RLC Branch3 : powerlib/Elements/Series RLC Branch  LConnTagsString=__new0  RConnTagsString=__new0  BranchType=L  Resistance=0  Inductance=0.152e-03  SetiL0=off  InitialCurrent=0  Capacitance=0  Setx0=off  InitialVoltage=0  Measurements=None
  Voltage Measurement1 : powerlib/Measurements/Voltage Measurement  PhasorSimulation=off  OutputType=Complex  PSBequivalent=0
  Voltage Measurement2 : powerlib/Measurements/Voltage Measurement  PhasorSimulation=off  OutputType=Complex  PSBequivalent=0
  Va : PMIOPort  Port=1  Side=Left
  Vin+ : PMIOPort  Port=2  Side=Left
  Vin- : PMIOPort  Port=3  Side=Left
  Vm : PMIOPort  Port=4  Side=Left
  wires:
  PWM Generator (DC-DC)/1 -> IGBT/Diode3/1
  Voltage Measurement1/1 -> Scope2/1
  Current Measurement2/1 -> Scope4/1
  D/1 -> PWM Generator (DC-DC)/1
  D1/1 -> PWM Generator (DC-DC)1/1
  Voltage Measurement2/1 -> Scope1/1
  PWM Generator (DC-DC)1/1 -> IGBT/Diode1/1
  Current Measurement1/1 -> Scope3/1
  connections:
  Series RLC Branch2/RConn1 -- Voltage Measurement2/LConn2 -- IGBT/Diode3/RConn1 -- Ground/LConn1 -- Voltage Measurement1/LConn2 -- CB1/RConn1 -- Vin-/RConn1 -- IGBT/Diode1/RConn1
  Current Measurement2/RConn1 -- Diode4/LConn1
  CB1/LConn1 -- Diode4/RConn1 -- Vm/RConn1 -- Voltage Measurement1/LConn1
  LB1/RConn1 -- Current Measurement2/LConn1 -- IGBT/Diode3/LConn1
  IGBT/Diode1/LConn1 -- Series RLC Branch3/LConn1 -- Vin+/RConn1 -- LB1/LConn1
  Diode1/RConn1 -- Series RLC Branch2/LConn1 -- Va/RConn1 -- Voltage Measurement2/LConn1
  Current Measurement1/RConn1 -- Diode1/LConn1
  Series RLC Branch3/RConn1 -- Current Measurement1/LConn1

== system bms_final_sims_06/Electrical system/DC Motor ==
  BL : Gain  Gain=0.1  SaturateOnIntegerOverflow=on  OutDataTypeStr=Inherit: Same as input  ParamDataTypeStr=Inherit: Same as input
  Bus Selector : BusSelector  OutputSignals=Speed wm (rad/s),Electrical torque Te (n m),Armature current ia (A),Field current if (A)
  DC_Motor : powerlib/Machines/DC Machine  PresetModel=No  MechanicalLoad=Torque TL  FieldType=Wound  ShowDetailedParameters=on  MeasurementBus=off  RLa="[ 0.6  0.012]"  RLf="[ 240  120]"  Laf=1.8  MachineConstant=Torque constant (N.m/A)  Ke=1.8  Kt=1.8  J=1  Bm=0  Tf=0  w0=1  Ifinit=1  TsPowergui=0  TsBlock=-1
  Demux1 : Demux
  Ef : powerlib/Electrical Sources/DC Voltage Source  Amplitude=Amplitude  Measurements=None
  Ground3 : powerlib/Elements/Ground  LConnTagsString=a
  Ia : Scope
  Scope : Scope  NumInputPorts=2
  Scope1 : Scope  NumInputPorts=2
  Te : Scope
  Terminator : Terminator
  w : Scope
  Vm : PMIOPort  Port=1  Side=Left
  wout : Outport
  wires:
  Demux1/1 -> BL/1, wout/1, w/1
  BL/1 -> DC_Motor/1
  Demux1/3 -> Terminator/1
  DC_Motor/1 -> Bus Selector/1, Demux1/1
  Demux1/4 -> Te/1
  Demux1/2 -> Ia/1
  Bus Selector/4 -> Scope/2  "<Field current if (A)>"
  Bus Selector/3 -> Scope/1  "<Armature current ia (A)>"
  Bus Selector/1 -> Scope1/1  "<Speed wm (rad/s)>"
  Bus Selector/2 -> Scope1/2  "<Electrical torque Te (n m)>"
  connections:
  DC_Motor/RConn1 -- Ground3/LConn1
  Ef/RConn1 -- DC_Motor/LConn2
  DC_Motor/RConn2 -- Ef/LConn1
  Vm/RConn1 -- DC_Motor/LConn1

== system bms_final_sims_06/Electrical system/Dashboard Test ==
  Total Fault Test : Subsystem

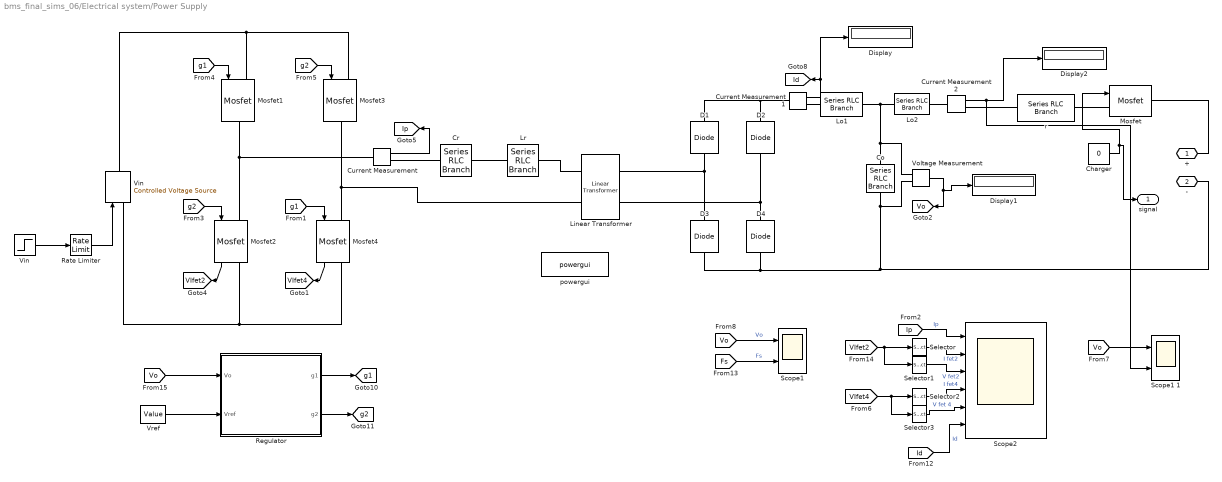
== system bms_final_sims_06/Electrical system/Power Supply ==
  "Charger " : Constant  Value=0
  Co : powerlib/Elements/Series RLC Branch  LConnTagsString=__new0  RConnTagsString=__new0  BranchType=C  Resistance=1e-4  Inductance=200e-6  SetiL0=off  InitialCurrent=0  Capacitance=Capacitance  Setx0=on  InitialVoltage=24  Measurements=None
  Cr : powerlib/Elements/Series RLC Branch  LConnTagsString=__new0  RConnTagsString=__new0  BranchType=C  Resistance=1e-4  Inductance=200e-6  SetiL0=off  InitialCurrent=0  Capacitance=160e-9  Setx0=off  InitialVoltage=40  Measurements=None
  Current Measurement : powerlib/Measurements/Current Measurement  PhasorSimulation=off  OutputType=Complex  PSBequivalent=0
  Current Measurement1 : powerlib/Measurements/Current Measurement  PhasorSimulation=off  OutputType=Complex  PSBequivalent=0
  Current Measurement2 : powerlib/Measurements/Current Measurement  PhasorSimulation=off  OutputType=Complex  PSBequivalent=0
  D{1..4} (4 alike) : powerlib/Power Electronics/Diode  Ron=1e-3  Lon=0  Vf=0.5  IC=0  UseSnubber=off  Rs=1e6  Cs=inf  Measurements=off
  Display : Display
  Display1 : Display
  Display2 : Display
  Linear Transformer : powerlib/Elements/Linear Transformer  UNITS=SI  NominalPower=[ 200 85e3 ]  winding1="[52   1e-2  75e-6]"  winding2="[6  1e-2  1.36e-6 ]"  ThreeWindings=off  winding3=[3.15e+05 0.7938 0.084225]  RmLm=[1e4 963e-6]  Measurements=None  DataType=on
  Lo1 : powerlib/Elements/Series RLC Branch  LConnTagsString=__new0  RConnTagsString=__new0  BranchType=L  Resistance=0.005  Inductance=Inductance  SetiL0=off  InitialCurrent=0  Capacitance=1e-6  Setx0=off  InitialVoltage=0  Measurements=None
  Lo2 : powerlib/Elements/Series RLC Branch  LConnTagsString=__new0  RConnTagsString=__new0  BranchType=L  Resistance=0.005  Inductance=Inductance1  SetiL0=off  InitialCurrent=0  Capacitance=1e-6  Setx0=off  InitialVoltage=0  Measurements=None
  Lr : powerlib/Elements/Series RLC Branch  LConnTagsString=__new0  RConnTagsString=__new0  BranchType=L  Resistance=1e-4  Inductance=37.5e-6  SetiL0=off  InitialCurrent=0  Capacitance=15e-9  Setx0=off  InitialVoltage=40  Measurements=None
  Mosfet : powerlib/Power Electronics/Mosfet  Ron=0.1  Lon=0  Rd=0.01  Vfd=0  IC=0  Rs=1e5  Cs=inf  Measurements=off
  Mosfet1 : powerlib/Power Electronics/Mosfet  Ron=1e-3  Lon=0  Rd=1e-3  Vfd=0  IC=0  Rs=1e6  Cs=inf  Measurements=off
  Mosfet2 : powerlib/Power Electronics/Mosfet  Ron=1e-3  Lon=0  Rd=1e-3  Vfd=0  IC=0  Rs=1e6  Cs=inf  Measurements=on
  Mosfet3 : powerlib/Power Electronics/Mosfet  Ron=1e-3  Lon=0  Rd=1e-3  Vfd=0  IC=0  Rs=1e6  Cs=inf  Measurements=off
  Mosfet4 : powerlib/Power Electronics/Mosfet  Ron=1e-3  Lon=0  Rd=1e-3  Vfd=0  IC=0  Rs=1e6  Cs=inf  Measurements=on
  Rate Limiter : RateLimiter  RisingSlewLimit=50e3  FallingSlewLimit=-50e3  SampleTimeMode=inherited  InitialCondition=390
  "Regulator " : Subsystem
  "Scope1 " : Scope  NumInputPorts=2
  Scope1 1 : Scope  NumInputPorts=2
  Scope2 : Scope  NumInputPorts=6
  Selector : Selector  InputPortWidth=2  IndexOptions=Index vector (dialog)  Indices=1  OutputSizes=1
  Selector1 : Selector  InputPortWidth=2  IndexOptions=Index vector (dialog)  Indices=2  OutputSizes=1
  Selector2 : Selector  InputPortWidth=2  IndexOptions=Index vector (dialog)  Indices=1  OutputSizes=1
  Selector3 : Selector  InputPortWidth=2  IndexOptions=Index vector (dialog)  Indices=2  OutputSizes=1
  Vin : Step  Time=0.004  Before=400  After=400  SampleTime=Ts_Control
  "Vin " : powerlib/Electrical Sources/Controlled Voltage Source  Initialize=on  Source_Type=DC  Amplitude=0  Phase=0  Frequency=0  Measurements=None
  Voltage Measurement : powerlib/Measurements/Voltage Measurement  PhasorSimulation=off  OutputType=Complex  PSBequivalent=0
  Vref : Constant  Value=Value
  powergui : powerlib/powergui  Priority=1  SimulationMode=Continuous  SampleTime=50e-6  frequency=60  Iterations=50  frequencyindice=0  Pbase=100e6  ErrMax=1e-4  UnitsV=kV  UnitsW=MW  buscounter=0  FunctionMessages=on  echomessages=off  EnableUseOfTLC=off  CurrentSourceSwitches=off  DisableSnubberDevices=off  DisableRonSwitches=off  DisableVfSwitches=off  DisplayEquations=off  SolverType=Tustin/Backward Euler (TBE)  Interpol=off  ExternalGateDelay=off  methode=off  Ts=100  x0status=blocks  SPID=on  SwTol=0  HookPort=off  RestoreLinks=warning  ResistiveCurrentMeasurement=off  Frange=[0:2:500]  Ylog=off  Xlog=on  ShowGrid=off  save=off  variable=ZData  structure=0  ZoomFFT=off  StartTime=0.0  cycles=1  DisplayStyle=1  fundamental=60  FreqAxis=off  MaxFrequency=1000  frequencyindicesteady=1  RmsSteady=1  display=off
  r : powerlib/Elements/Series RLC Branch  LConnTagsString=__new0  RConnTagsString=__new0  BranchType=R  Resistance=0.001  Inductance=1e-3  SetiL0=off  InitialCurrent=0  Capacitance=1e-6  Setx0=off  InitialVoltage=0  Measurements=None
  + : PMIOPort  Port=1  Side=Left
  - : PMIOPort  Port=2  Side=Left
  signal : Outport
  tag scope: Id=global, Ip=global, VIfet2=global, VIfet4=global, Vo=global, g1=global, g2=global
  wires:
  [g2] -> Mosfet2/1
  Current Measurement/1 -> [Ip]
  [g1] -> Mosfet1/1
  Voltage Measurement/1 -> Display1/1, [Vo]
  [Ip] -> Scope2/1  "Ip"
  Selector1/1 -> Scope2/3  "V fet2"
  [Vo] -> "Regulator "/1(Vo)
  "Regulator "/2(g2) -> [g2]
  Vin/1 -> Rate Limiter/1
  Selector3/1 -> Scope2/5  "V fet 4"
  [Fs] -> "Scope1 "/2  "Fs"
  [Id] -> Scope2/6  "Id"
  "Regulator "/1(g1) -> [g1]
  Selector2/1 -> Scope2/4  "I fet4"
  Selector/1 -> Scope2/2  "I fet2"
  [g1] -> Mosfet4/1
  Rate Limiter/1 -> "Vin "/1
  Mosfet2/1 -> [VIfet2]
  Mosfet4/1 -> [VIfet4]
  Vref/1 -> "Regulator "/2(Vref)
  [g2] -> Mosfet3/1
  Current Measurement1/1 -> Display/1, [Id]
  [VIfet2] -> Selector1/1, Selector/1
  [VIfet4] -> Selector3/1, Selector2/1
  [Vo] -> "Scope1 "/1  "Vo"
  "Charger "/1 -> signal/1, Mosfet/1
  [Vo] -> Scope1 1/1
  Current Measurement2/1 -> Scope1 1/2, Display2/1
  connections:
  Mosfet2/LConn1 -- Current Measurement/LConn1 -- Mosfet1/RConn1
  "Vin "/RConn1 -- Mosfet3/LConn1 -- Mosfet1/LConn1
  Cr/LConn1 -- Current Measurement/RConn1
  Linear Transformer/RConn2 -- D4/RConn1 -- D2/LConn1
  Co/RConn1 -- Voltage Measurement/LConn2 -- -/RConn1 -- D4/LConn1 -- D3/LConn1
  "Vin "/LConn1 -- Mosfet4/RConn1 -- Mosfet2/RConn1
  Linear Transformer/RConn1 -- D3/RConn1 -- D1/LConn1
  Voltage Measurement/LConn1 -- Lo2/LConn1 -- Lo1/RConn1 -- Co/LConn1
  Lr/LConn1 -- Cr/RConn1
  Mosfet4/LConn1 -- Linear Transformer/LConn2 -- Mosfet3/RConn1
  Lr/RConn1 -- Linear Transformer/LConn1
  D1/RConn1 -- D2/RConn1 -- Current Measurement1/LConn1
  Mosfet/RConn1 -- +/RConn1
  Lo1/LConn1 -- Current Measurement1/RConn1
  Lo2/RConn1 -- Current Measurement2/LConn1
  r/RConn1 -- Mosfet/LConn1
  r/LConn1 -- Current Measurement2/RConn1

== system bms_final_sims_06/Electrical system/Battery Management system/ function ==
  Ib : Inport
  SocB : Inport  Port=2
  wm : Inport  Port=3
  MATLAB Function : MATLAB Function  TreatAsAtomicUnit=on
  MATLAB Function1 : MATLAB Function  TreatAsAtomicUnit=on
  MATLAB Function2 : MATLAB Function  TreatAsAtomicUnit=on
  Range : Outport
  SoH : Outport  Port=2
  wires:
  MATLAB Function/1(soh) -> SoH/1
  Ib/1 -> MATLAB Function1/1(I)
  wm/1 -> MATLAB Function1/2(w)
  MATLAB Function2/1(R) -> Range/1
  SocB/1 -> MATLAB Function/1(soc), MATLAB Function2/2(S)
  MATLAB Function1/1(Iavg) -> MATLAB Function2/1(Iavg)
  MATLAB Function1/2(wavg) -> MATLAB Function2/3(wavg)

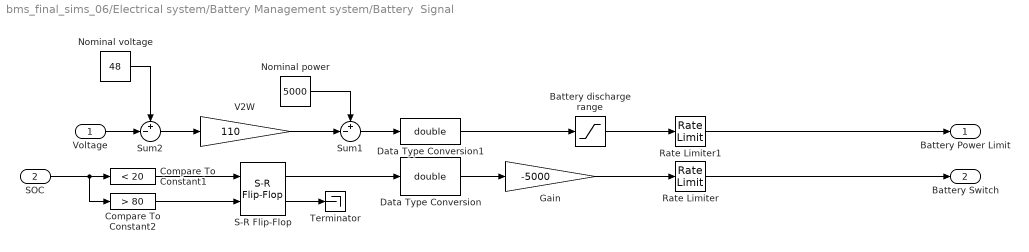
== system bms_final_sims_06/Electrical system/Battery Management system/Battery  Signal ==
  Voltage : Inport
  SOC : Inport  Port=2
  Battery discharge range : Saturate  UpperLimit=5000  LowerLimit=0
  Compare To Constant1 : simulink/Logic and Bit Operations/Compare To Constant  relop=<  const=20  OutDataTypeStr=boolean
  Compare To Constant2 : simulink/Logic and Bit Operations/Compare To Constant  relop=>  const=80  OutDataTypeStr=boolean
  Data Type Conversion : DataTypeConversion  OutDataTypeStr=double  SampleTime=0
  Data Type Conversion1 : DataTypeConversion  OutDataTypeStr=double  SampleTime=0
  Gain : Gain  Gain=-5000
  Nominal power : Constant  Value=5000
  Nominal voltage : Constant  Value=48
  Rate Limiter : RateLimiter  RisingSlewLimit=10000  FallingSlewLimit=-10000  SampleTimeMode=inherited
  Rate Limiter1 : RateLimiter  RisingSlewLimit=50000  FallingSlewLimit=-50000  SampleTimeMode=inherited
  S-R Flip-Flop : simulink_extras/Flip Flops/S-R Flip-Flop  initial_condition=0
  Sum1 : Sum  Inputs=+-|
  Sum2 : Sum  Inputs=+-|
  Terminator : Terminator
  V2W : Gain  Gain=110
  "Battery Power Limit " : Outport
  Battery Switch : Outport  Port=2
  wires:
  Compare To Constant2/1 -> S-R Flip-Flop/2
  Compare To Constant1/1 -> S-R Flip-Flop/1
  Gain/1 -> Rate Limiter/1
  Battery discharge range/1 -> Rate Limiter1/1
  S-R Flip-Flop/1 -> Data Type Conversion/1
  Rate Limiter/1 -> Battery Switch/1
  Nominal voltage/1 -> Sum2/1
  Rate Limiter1/1 -> "Battery Power Limit "/1
  V2W/1 -> Sum1/2
  Data Type Conversion/1 -> Gain/1
  Data Type Conversion1/1 -> Battery discharge range/1
  S-R Flip-Flop/2 -> Terminator/1
  Nominal power/1 -> Sum1/1
  Sum1/1 -> Data Type Conversion1/1
  Sum2/1 -> V2W/1
  Voltage/1 -> Sum2/2
  SOC/1 -> Compare To Constant1/1, Compare To Constant2/1

== system bms_final_sims_06/Electrical system/Battery Management system/Break Unit ==
  Ir : Inport
  Vr : Inport  Port=2
  Battery Temp : Inport  Port=3
  "cont Status " : Inport  Port=4
  Circuit Braker Signal : Subsystem
  Ground : Ground
  Sensors : Subsystem
  Out1 : Outport
  wires:
  Circuit Braker Signal/1(C) -> Out1/1
  Sensors/3(Ex Fault3) -> Circuit Braker Signal/3(Ex Fault3)
  Sensors/1(Ex Fault1) -> Circuit Braker Signal/1(Ex Fault1)
  Sensors/2(Ex Fault2) -> Circuit Braker Signal/2(Ex Fault2)
  Ir/1 -> Sensors/1(Ir)
  Vr/1 -> Sensors/2(Vr)
  Battery Temp/1 -> Sensors/3(Battery Temp)
  Ground/1 -> Circuit Braker Signal/5(Emergency Trip)
  Sensors/4(Ex Fault4) -> Circuit Braker Signal/4(Ex Fault4)
  "cont Status "/1 -> Circuit Braker Signal/6(CS)
